simulink model "INUSimulator"  (Simulink 6.6)
settings: Solver=ode45  StartTime=0.0  StopTime=10.0  RelTol=1e-3
undefined symbols (not defined in the file or in its folder): DiscIntNeverNeededParam
settings Model: Creator=dgitz  LastModifiedBy=dgitz

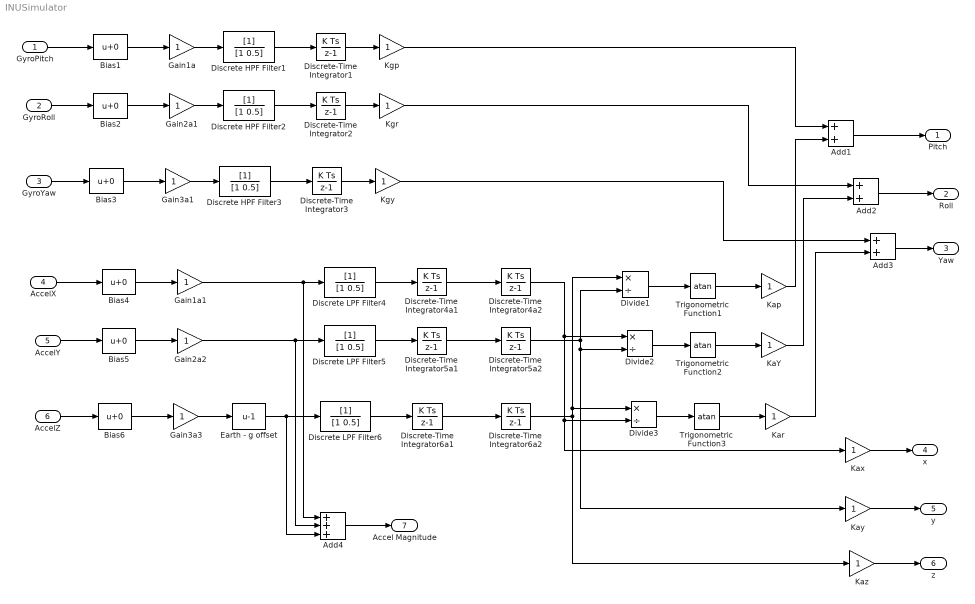
== system INUSimulator ==
  GyroPitch : Inport
  GyroRoll : Inport  Port=2
  GyroYaw : Inport  Port=3
  AccelX : Inport  Port=4
  AccelY : Inport  Port=5
  AccelZ : Inport  Port=6
  Add1 : Sum  OutScaling=2^-10
  Add2 : Sum  OutScaling=2^-10
  Add3 : Sum  OutScaling=2^-10
  Add4 : Sum  Inputs=+++  OutScaling=2^-10
  Bias{1..6} (6 alike) : Bias
  Discrete HPF Filter1 : DiscreteFilter  Denominator=[1 0.5]
  Discrete HPF Filter2 : DiscreteFilter  Denominator=[1 0.5]
  Discrete HPF Filter3 : DiscreteFilter  Denominator=[1 0.5]
  Discrete LPF Filter4 : DiscreteFilter  Denominator=[1 0.5]
  Discrete LPF Filter5 : DiscreteFilter  Denominator=[1 0.5]
  Discrete LPF Filter6 : DiscreteFilter  Denominator=[1 0.5]
  Discrete-Time Integrator1 : DiscreteIntegrator  LimitOutput=on  UpperSaturationLimit=360  LowerSaturationLimit=0  ICPrevOutput=DiscIntNeverNeededParam  ICPrevScaledInput=DiscIntNeverNeededParam
  Discrete-Time Integrator2 : DiscreteIntegrator  LimitOutput=on  UpperSaturationLimit=360  LowerSaturationLimit=0  ICPrevOutput=DiscIntNeverNeededParam  ICPrevScaledInput=DiscIntNeverNeededParam
  Discrete-Time Integrator3 : DiscreteIntegrator  SampleTime=-1  LimitOutput=on  UpperSaturationLimit=360  LowerSaturationLimit=0  ICPrevOutput=DiscIntNeverNeededParam  ICPrevScaledInput=DiscIntNeverNeededParam
  Discrete-Time Integrator4a1 : DiscreteIntegrator  LimitOutput=on  UpperSaturationLimit=360  LowerSaturationLimit=0  ICPrevOutput=DiscIntNeverNeededParam  ICPrevScaledInput=DiscIntNeverNeededParam
  Discrete-Time Integrator4a2 : DiscreteIntegrator  LimitOutput=on  UpperSaturationLimit=360  LowerSaturationLimit=0  ICPrevOutput=DiscIntNeverNeededParam  ICPrevScaledInput=DiscIntNeverNeededParam
  Discrete-Time Integrator5a1 : DiscreteIntegrator  LimitOutput=on  UpperSaturationLimit=360  LowerSaturationLimit=0  ICPrevOutput=DiscIntNeverNeededParam  ICPrevScaledInput=DiscIntNeverNeededParam
  Discrete-Time Integrator5a2 : DiscreteIntegrator  LimitOutput=on  UpperSaturationLimit=360  LowerSaturationLimit=0  ICPrevOutput=DiscIntNeverNeededParam  ICPrevScaledInput=DiscIntNeverNeededParam
  Discrete-Time Integrator6a1 : DiscreteIntegrator  SampleTime=-1  LimitOutput=on  UpperSaturationLimit=360  LowerSaturationLimit=0  ICPrevOutput=DiscIntNeverNeededParam  ICPrevScaledInput=DiscIntNeverNeededParam
  Discrete-Time Integrator6a2 : DiscreteIntegrator  SampleTime=-1  LimitOutput=on  UpperSaturationLimit=360  LowerSaturationLimit=0  ICPrevOutput=DiscIntNeverNeededParam  ICPrevScaledInput=DiscIntNeverNeededParam
  Divide1 : Product  Inputs=*/  OutScaling=2^-10
  Divide2 : Product  Inputs=*/  OutScaling=2^-10
  Divide3 : Product  Inputs=*/  OutScaling=2^-10
  Earth - g offset : Bias  Bias=-1
  Gain1a : Gain
  Gain1a1 : Gain
  Gain2a1 : Gain
  Gain2a2 : Gain
  Gain3a1 : Gain
  Gain3a3 : Gain
  KaY : Gain
  Kap : Gain
  Kar : Gain
  Kax : Gain
  Kay : Gain
  Kaz : Gain
  Kgp : Gain
  Kgr : Gain
  Kgy : Gain
  Trigonometric Function1 : Trigonometry  Operator=atan
  Trigonometric Function2 : Trigonometry  Operator=atan
  Trigonometric Function3 : Trigonometry  Operator=atan
  Pitch : Outport
  Roll : Outport  Port=2
  Yaw : Outport  Port=3
  x : Outport  Port=4
  y : Outport  Port=5
  z : Outport  Port=6
  Accel Magnitude : Outport  Port=7
  wires:
  GyroPitch/1 -> Bias1/1
  Bias1/1 -> Gain1a/1
  Gain1a/1 -> Discrete HPF Filter1/1
  Discrete HPF Filter1/1 -> Discrete-Time Integrator1/1
  Discrete-Time Integrator1/1 -> Kgp/1
  Bias2/1 -> Gain2a1/1
  Gain2a1/1 -> Discrete HPF Filter2/1
  Discrete HPF Filter2/1 -> Discrete-Time Integrator2/1
  Discrete-Time Integrator2/1 -> Kgr/1
  Bias3/1 -> Gain3a1/1
  Gain3a1/1 -> Discrete HPF Filter3/1
  Discrete HPF Filter3/1 -> Discrete-Time Integrator3/1
  Discrete-Time Integrator3/1 -> Kgy/1
  GyroRoll/1 -> Bias2/1
  GyroYaw/1 -> Bias3/1
  Bias4/1 -> Gain1a1/1
  Bias5/1 -> Gain2a2/1
  Bias6/1 -> Gain3a3/1
  AccelX/1 -> Bias4/1
  AccelY/1 -> Bias5/1
  AccelZ/1 -> Bias6/1
  Gain3a3/1 -> Earth - g offset/1
  Discrete LPF Filter4/1 -> Discrete-Time Integrator4a1/1
  Discrete LPF Filter5/1 -> Discrete-Time Integrator5a1/1
  Discrete LPF Filter6/1 -> Discrete-Time Integrator6a1/1
  Gain1a1/1 -> Discrete LPF Filter4/1, Add4/1
  Gain2a2/1 -> Discrete LPF Filter5/1, Add4/2
  Earth - g offset/1 -> Discrete LPF Filter6/1, Add4/3
  Discrete-Time Integrator4a1/1 -> Discrete-Time Integrator4a2/1
  Discrete-Time Integrator5a1/1 -> Discrete-Time Integrator5a2/1
  Discrete-Time Integrator6a1/1 -> Discrete-Time Integrator6a2/1
  Divide1/1 -> Trigonometric Function1/1
  Divide2/1 -> Trigonometric Function2/1
  Divide3/1 -> Trigonometric Function3/1
  Discrete-Time Integrator6a2/1 -> Divide1/1, Divide3/1, Kaz/1
  Discrete-Time Integrator5a2/1 -> Divide1/2, Divide2/2, Kay/1
  Discrete-Time Integrator4a2/1 -> Divide2/1, Divide3/2, Kax/1
  Trigonometric Function1/1 -> Kap/1
  Trigonometric Function2/1 -> KaY/1
  Trigonometric Function3/1 -> Kar/1
  Kgp/1 -> Add1/1
  Kap/1 -> Add1/2
  Kgr/1 -> Add2/1
  KaY/1 -> Add2/2
  Kar/1 -> Add3/2
  Kgy/1 -> Add3/1
  Add3/1 -> Yaw/1
  Add2/1 -> Roll/1
  Add1/1 -> Pitch/1
  Kax/1 -> x/1
  Kay/1 -> y/1
  Kaz/1 -> z/1
  Add4/1 -> Accel Magnitude/1
